simulink model "altitudine_correction"  (R2020a)
settings: Solver=VariableStepAuto  StartTime=0.0  StopTime=10.0  RelTol=1e-3
libraries: simulink_extras x3
settings Model: Creator=rpogl  LastModifiedBy=rpogl

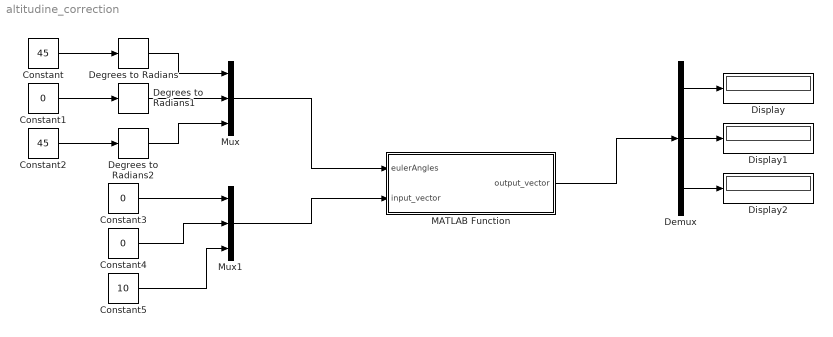
== system altitudine_correction ==
  Constant : Constant  Value=45
  Constant1 : Constant  Value=0
  Constant2 : Constant  Value=45
  Constant3 : Constant  Value=0
  Constant4 : Constant  Value=0
  Constant5 : Constant  Value=10
  Degrees to Radians : simulink_extras/Transformations/Degrees to Radians
  Degrees to Radians1 : simulink_extras/Transformations/Degrees to Radians
  Degrees to Radians2 : simulink_extras/Transformations/Degrees to Radians
  Demux : Demux  Outputs=3
  Display : Display
  Display1 : Display
  Display2 : Display
  MATLAB Function : MATLAB Function  TreatAsAtomicUnit=on
  Mux : Mux  Inputs=3
  Mux1 : Mux  Inputs=3
  wires:
  Mux1/1 -> MATLAB Function/2(input_vector)
  Mux/1 -> MATLAB Function/1(eulerAngles)
  Constant/1 -> Degrees to Radians/1
  Constant1/1 -> Degrees to Radians1/1
  Constant2/1 -> Degrees to Radians2/1
  Constant3/1 -> Mux1/1
  Constant4/1 -> Mux1/2
  Constant5/1 -> Mux1/3
  MATLAB Function/1(output_vector) -> Demux/1
  Degrees to Radians/1 -> Mux/1
  Degrees to Radians1/1 -> Mux/2
  Degrees to Radians2/1 -> Mux/3
  Demux/2 -> Display1/1
  Demux/1 -> Display/1
  Demux/3 -> Display2/1

== matlab function altitudine_correction/MATLAB Function ==
  data: eulerAngles input; output_vector output; input_vector input
function output_vector = fcn(eulerAngles , input_vector)

phi = eulerAngles(1);
theta = eulerAngles(2);
psi = eulerAngles(3);

Rx = [1 0 0; 0 cos(phi) -sin(phi); 0 sin(phi) cos(phi)];
Ry = [cos(theta) 0 sin(theta); 0 1 0; -sin(theta) 0 cos(theta)];
Rz = [cos(psi) -sin(psi) 0; sin(psi) cos(psi) 0; 0 0 1];

R = Rz * Ry * Rx;

output_vector = R * input_vector;
